simulink model "e3"  (R2014b)
settings: Solver=ode45  StartTime=0.0  StopTime=10.0  RelTol=1e-3
settings Model: Creator=Administrator  LastModifiedBy=Administrator

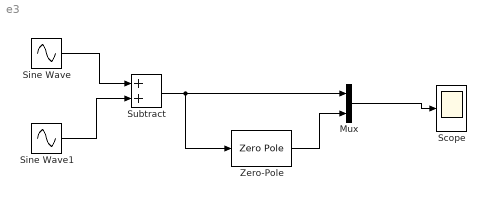
== system e3 ==
  Mux : Mux  Inputs=2
  Scope : Scope
      settings: TimeRange=0.5  YMin=-2  YMax=2
  Sine Wave : Sin  SampleTime=0
  Sine Wave1 : Sin  Frequency=100  SampleTime=0
  Subtract : Sum
  Zero-Pole : ZeroPole  Zeros=[0]  Poles=[-200*pi]  Gain=[6.4]
  wires:
  Sine Wave/1 -> Subtract/1
  Sine Wave1/1 -> Subtract/2
  Subtract/1 -> Zero-Pole/1, Mux/1
  Mux/1 -> Scope/1
  Zero-Pole/1 -> Mux/2
